simulink model "nonlinearFinal"  (R2023b)
settings: Solver=VariableStepAuto  StartTime=0.0  StopTime=10.0  RelTol=1e-3
undefined symbols (not defined in the file or in its folder): g, h, Ix, Iy, Iz, Kt, l, m
settings Model: Creator=lenovo  LastModifiedBy=artin
settings DebuggingCC: UnconnectedInputMsg=warning  UnconnectedOutputMsg=warning  UnconnectedLineMsg=warning
settings ModelReferenceCC: EnableRefExpFcnMdlSchedulingChecks=on
settings RTWCC: DLArmComputeVersion=19.05

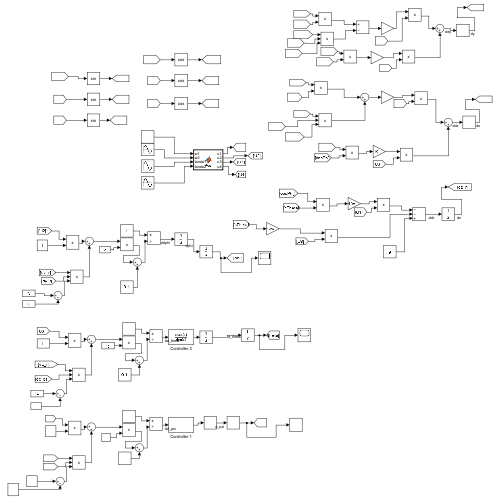
[thumbnail: Simulink's stored preview of the top-level diagram]
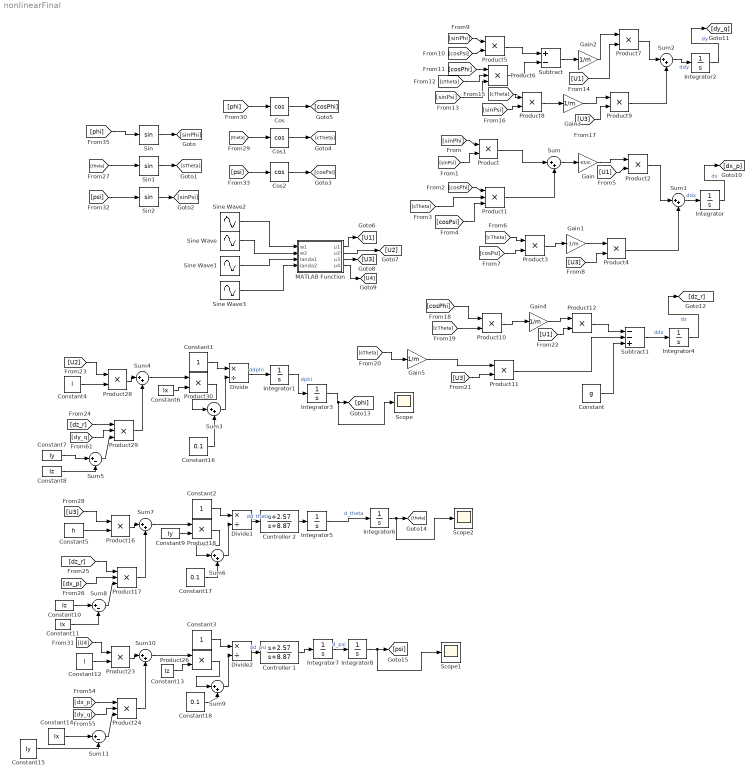
== system nonlinearFinal ==
  Constant : Constant  Value=g
  Constant1 : Constant
  Constant10 : Constant  Value=Iz
  Constant11 : Constant  Value=Ix
  Constant12 : Constant  Value=l
  Constant13 : Constant  Value=Iz
  Constant14 : Constant  Value=Ix
  Constant15 : Constant  Value=Iy
  Constant16 : Constant  Value=0.1
  Constant17 : Constant  Value=0.1
  Constant18 : Constant  Value=0.1
  Constant2 : Constant
  Constant3 : Constant
  Constant4 : Constant  Value=l
  Constant5 : Constant  Value=h
  Constant6 : Constant  Value=Ix
  Constant7 : Constant  Value=Iy
  Constant8 : Constant  Value=Iz
  Constant9 : Constant  Value=Iy
  Controller 1 : TransferFcn  Numerator=[1 2.57]  Denominator=[1 8.87]
  Controller 2 : TransferFcn  Numerator=[1 2.57]  Denominator=[1 8.87]
  Cos : Trigonometry  Operator=cos
  Cos1 : Trigonometry  Operator=cos
  Cos2 : Trigonometry  Operator=cos
  Divide : Product  Inputs=*/
  Divide1 : Product  Inputs=*/
  Divide2 : Product  Inputs=*/
  Gain : Gain  Gain=-Kt/m
  Gain1 : Gain  Gain=-1/m
  Gain{2..5} (4 alike) : Gain  Gain=1/m
  Integrator{,1..8} (9 alike) : Integrator
  MATLAB Function : MATLAB Function  TreatAsAtomicUnit=on
  Product{,2..5,7..12,16,18,23,26,28,30} (17 alike) : Product
  Product{1,6,17,24,29} (5 alike) : Product  Inputs=3
  Scope : Scope
  Scope1 : Scope
  Scope2 : Scope
  Sin : Trigonometry
  Sin1 : Trigonometry
  Sin2 : Trigonometry
  Sine Wave{,1..3} (4 alike) : Sin  SampleTime=0
  Subtract : Sum  Inputs=+-
  Subtract1 : Sum  Inputs=--+
  Sum{,1..4,6..7,9..10} (9 alike) : Sum  Inputs=|++
  Sum11 : Sum  Inputs=|+-
  Sum5 : Sum  Inputs=|+-
  Sum8 : Sum  Inputs=|+-
  wires:
  Sin1/1 -> [sTheta]
  Sin2/1 -> [sinPsi]
  Cos/1 -> [cosPhi]
  Cos1/1 -> [cTheta]
  Cos2/1 -> [cosPsi]
  [sinPhi] -> Product/1
  [sinPsi] -> Product/2
  [cosPhi] -> Product1/1
  [sTheta] -> Product1/2
  [cosPsi] -> Product1/3
  Product1/1 -> Sum/2
  Product/1 -> Sum/1
  Sum/1 -> Gain/1
  Gain/1 -> Product2/1
  MATLAB Function/1(u1) -> [U1]
  MATLAB Function/2(u2) -> [U2]
  MATLAB Function/3(u3) -> [U3]
  MATLAB Function/4(u4) -> [U4]
  [U1] -> Product2/2
  Sin/1 -> [sinPhi]
  [cTheta] -> Product3/1
  [cosPsi] -> Product3/2
  Product3/1 -> Gain1/1
  Gain1/1 -> Product4/1
  [U3] -> Product4/2
  Product2/1 -> Sum1/1
  Product4/1 -> Sum1/2
  Sum1/1 -> Integrator/1  "ddx"
  Integrator/1 -> [dx_p]  "dx"
  [sinPhi] -> Product5/1
  [cosPsi] -> Product5/2
  [cosPhi] -> Product6/1
  [sTheta] -> Product6/2
  [sinPsi] -> Product6/3
  Product5/1 -> Subtract/1
  Product6/1 -> Subtract/2
  Subtract/1 -> Gain2/1
  Gain2/1 -> Product7/1
  [U1] -> Product7/2
  [cTheta] -> Product8/1
  [sinPsi] -> Product8/2
  Product8/1 -> Gain3/1
  Gain3/1 -> Product9/1
  [U3] -> Product9/2
  Product7/1 -> Sum2/1
  Product9/1 -> Sum2/2
  Sum2/1 -> Integrator2/1  "ddy"
  Integrator2/1 -> [dy_q]  "dy"
  [cosPhi] -> Product10/1
  [cTheta] -> Product10/2
  Product10/1 -> Gain4/1
  [U3] -> Product11/2
  Gain5/1 -> Product11/1
  [sTheta] -> Gain5/1
  Gain4/1 -> Product12/1
  [U1] -> Product12/2
  Product12/1 -> Subtract1/1
  Product11/1 -> Subtract1/2
  Constant/1 -> Subtract1/3
  Subtract1/1 -> Integrator4/1  "ddz"
  Integrator4/1 -> [dz_r]  "dz"
  Sum10/1 -> Product26/1
  [dx_p] -> Product24/1
  Divide/1 -> Integrator1/1  "ddphi"
  Product29/1 -> Sum4/2
  Constant12/1 -> Product23/2
  Sum11/1 -> Product24/3
  Constant13/1 -> Product26/2
  [dy_q] -> Product24/2
  Product24/1 -> Sum10/2
  Product23/1 -> Sum10/1
  Constant1/1 -> Divide/1
  Product28/1 -> Sum4/1
  Constant14/1 -> Sum11/1
  Constant3/1 -> Divide2/1
  Constant8/1 -> Sum5/2
  Sum8/1 -> Product17/3
  Constant5/1 -> Product16/2
  Constant9/1 -> Product18/2
  Product16/1 -> Sum7/1
  Product17/1 -> Sum7/2
  Constant10/1 -> Sum8/1
  Constant2/1 -> Divide1/1
  Constant7/1 -> Sum5/1
  Constant15/1 -> Sum11/2
  Sum7/1 -> Product18/1
  Constant6/1 -> Product30/2
  Sum5/1 -> Product29/3
  Constant4/1 -> Product28/2
  [dy_q] -> Product29/2
  Sum4/1 -> Product30/1
  [dz_r] -> Product29/1
  [U2] -> Product28/1
  Integrator1/1 -> Integrator3/1  "dphi"
  Integrator3/1 -> Scope/1, [phi]
  [phi] -> Sin/1
  [U3] -> Product16/1
  Constant11/1 -> Sum8/2
  [dz_r] -> Product17/1
  [dx_p] -> Product17/2
  Integrator5/1 -> Integrator6/1  "d_theta"
  Integrator6/1 -> Scope2/1, [theta]
  [theta] -> Sin1/1
  [phi] -> Cos/1
  [theta] -> Cos1/1
  [U4] -> Product23/1
  Integrator7/1 -> Integrator8/1  "d_psi"
  Integrator8/1 -> Scope1/1, [psi]
  [psi] -> Sin2/1
  [psi] -> Cos2/1
  Sine Wave2/1 -> MATLAB Function/1(w1)
  Sine Wave/1 -> MATLAB Function/2(w2)
  Sine Wave1/1 -> MATLAB Function/3(landa1)
  Sine Wave3/1 -> MATLAB Function/4(landa2)
  Product30/1 -> Sum3/1
  Sum3/1 -> Divide/2
  Constant16/1 -> Sum3/2
  Constant17/1 -> Sum6/2
  Product18/1 -> Sum6/1
  Sum6/1 -> Divide1/2
  Constant18/1 -> Sum9/2
  Product26/1 -> Sum9/1
  Sum9/1 -> Divide2/2
  Divide2/1 -> Controller 1/1  "dd_psi"
  Controller 1/1 -> Integrator7/1
  Divide1/1 -> Controller 2/1  "dd_theta"
  Controller 2/1 -> Integrator5/1

== matlab function nonlinearFinal/MATLAB Function ==
  data: w1 input; u1 output; w2 input; landa1 input; landa2 input; u2 output; u3 output; u4 output
function [u1,u2,u3,u4] = fcn(w1,w2,landa1,landa2)
%these constants must be evaluated in order for the SIMULINK model to work
 
g=9.81;
h=0.085;
l=0.175;
Kt=6.46;
m=0.87;
Ix=0.0043;
Iy=0.0142;
Iz=0.0176;

u1=Kt*(w1*w1*cos(landa1)+w2*w2*cos(landa2));
u2=Kt*(w1*w1*cos(landa1)-w2*w2*cos(landa2));
u3=Kt*(w1*w1*sin(landa1)+w2*w2*sin(landa2));
u4=Kt*(w1*w1*sin(landa1)-w2*w2*sin(landa2));
